simulink model "Rakete2"  (Simulink 7.9)
settings: Solver=ode45  StartTime=0.0  StopTime=600  RelTol=1e-3
settings Model: Creator=karo  LastModifiedBy=karo

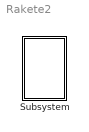
== system Rakete2 ==
  Subsystem : Subsystem  mask{m1_leer=500, m2_leer=1000, St1_Treibstoff=4000, St2_Treibstoff=1500, Durchsatz_1=20, Durchsatz_2=15, SchubProDurchsatz=4000}

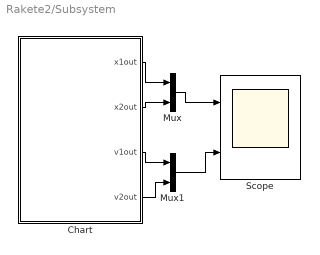
== system Rakete2/Subsystem ==
  Chart : Stateflow chart  TreatAsAtomicUnit=on
  Mux : Mux  Inputs=2
  Mux1 : Mux  Inputs=2
  Scope : Scope  NumInputPorts=2
      settings: YMin=-5~-5  YMax=5~5
  wires:
  Mux/1 -> Scope/1
  Chart/3(v1out) -> Mux1/1
  Chart/4(v2out) -> Mux1/2
  Mux1/1 -> Scope/2
  Chart/1(x1out) -> Mux/1
  Chart/2(x2out) -> Mux/2

== stateflow chart Subsystem/Chart ==
  settings: updateMethod=CONTINUOUS
  state StufenGemeinsam
    during:
    // Derivatives
    [v1_dot, v2_dot] = Acc1();
    x1_dot = v1;
    x2_dot = v2;
    m1_dot = -Durchsatz_1;
    m2_dot = 0;
    //Output
    x1out = x1;
    x2out = x2;
    v1out = v1;
    v2out = v2;
  state StufenGetrennt
    during:
    //Derivatives
    [v1_dot, v2_dot] = Acc2();
    x1_dot = v1;
    x2_dot = v2;
    m1_dot = 0;
    m2_dot = -Durchsatz_2;
    // Output
    x1out = x1;
    v1out = v1;
    x2out = x2;
    v2out = v2;
  state Stufe2Ausgebrannt
    during:
    //Derivatives
    [v1_dot, v2_dot] = Acc3();
    x1_dot = v1;
    x2_dot = v2;
    m1_dot = 0;
    m2_dot = 0;
    // Output
    x1out = x1;
    v1out = v1;
    x2out = x2;
    v2out = v2;
  (default) -> StufenGemeinsam : {Init();}
  StufenGemeinsam -> StufenGetrennt : [m1 <= m1_leer]
      | {m1 = m1_leer}
  StufenGetrennt -> Stufe2Ausgebrannt : [m2 <= m2_leer]
      | {m2 = m2_leer}
  data: a1 function_output double; a2 function_output double; a1 function_output double; a2 function_output double; a1 function_output double; a2 function_output double; m1_leer parameter double; m2_leer parameter double; St2_Treibstoff parameter double; Durchsatz_1 parameter double; Durchsatz_2 parameter double; SchubProDurchsatz parameter double; x1 local double; v1 local double; St1_Treibstoff parameter double; x2 local double; v2 local double; m1 local double; m2 local double; x1out output double; x2out output double; v1out output double; v2out output double; Erdmasse constant double =5.9736*10^24; Erdradius constant double =6378000; G constant double =66.743*10^-12
  data x1 settings: updateMethod=SF_CONTINUOUS_TIME_DATA
  data v1 settings: updateMethod=SF_CONTINUOUS_TIME_DATA
  data x2 settings: updateMethod=SF_CONTINUOUS_TIME_DATA
  data v2 settings: updateMethod=SF_CONTINUOUS_TIME_DATA
  data m1 settings: updateMethod=SF_CONTINUOUS_TIME_DATA
  data m2 settings: updateMethod=SF_CONTINUOUS_TIME_DATA
  function Init:
    | function Init
    |     x1 = 0;
    |     v1 = 0;
    |     x2 = 0;
    |     v2 = 0;
    |     m1 = m1_leer + St1_Treibstoff;
    |     m2 = m2_leer + St2_Treibstoff;
    | end
  function [a1, a2] = Acc1:
    | function [a1, a2] = Acc1
    |     Schubkraft = Durchsatz_1 * SchubProDurchsatz;
    |     mRakete = m1 + m2;
    |     r = Erdradius + x1;
    |     FS = (G * mRakete * Erdmasse) / (r^2);
    |     % aus summe F = m * a -->
    |     a1 = (Schubkraft - FS) / (mRakete);
    |     a2 = a1;
    | end
  function [a1, a2] = Acc2:
    | function [a1, a2] = Acc2
    | % 1. Stufe bereits ausgebrannt
    |     Schubkraft = Durchsatz_2 * SchubProDurchsatz;
    |     
    |     r1 = Erdradius + x1;
    |     r2 = Erdradius + x2;
    |     
    |     FS1 = (G * m1 * Erdmasse) / (r1^2);
    |     FS2 = (G * m2 * Erdmasse) / (r2^2);
    |     % aus summe F = m * a -->
    |     a1 = (-FS1) / (m1);
    |     a2 = (Schubkraft - FS2) / m2;
    | end
  function [a1, a2] = Acc3:
    | function [a1, a2] = Acc3
    | % beider Stufen bereits ausgebrannt    
    |     r1 = Erdradius + x1;
    |     r2 = Erdradius + x2;
    |     
    |     FS1 = (G * m1 * Erdmasse) / (r1^2);
    |     FS2 = (G * m2 * Erdmasse) / (r2^2);
    |     % aus summe F = m * a -->
    |     a1 = (-FS1) / (m1);
    |     a2 = (-FS2) / m2;
    | end
